simulink subsystem "Point2SHP"  (R2023a)
settings: Solver=VariableStepAuto  StartTime=0.0  StopTime=10.0  RelTol=1e-3
undefined symbols (not defined in the file): magnitude
settings Model: Creator=bjmyn  LastModifiedBy=bjmyn

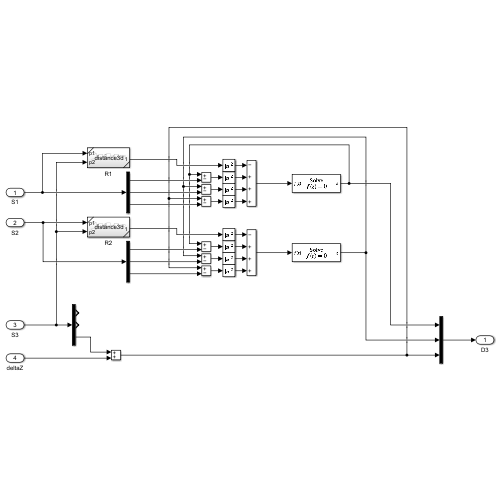
[thumbnail: Simulink's stored preview of the top-level diagram]
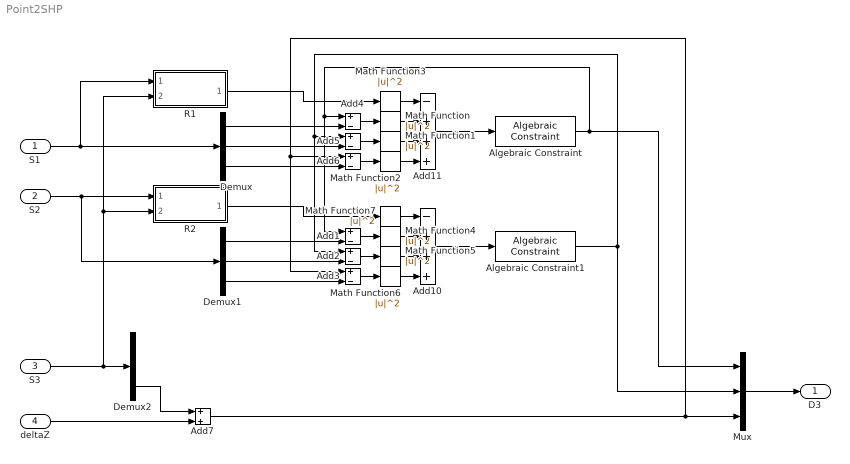
== system Point2SHP ==
  S1 : Inport
  S2 : Inport  Port=2
  S3 : Inport  Port=3
  deltaZ : Inport  Port=4
  Add{1..6} (6 alike) : Sum  Inputs=+-
  Add10 : Sum  Inputs=-+++
  Add11 : Sum  Inputs=-+++
  Add7 : Sum
  Algebraic Constraint : AlgebraicConstraint
  Algebraic Constraint1 : AlgebraicConstraint  InitialGuess=460
  Demux : Demux  Outputs=3
  Demux1 : Demux  Outputs=3
  Demux2 : Demux  Outputs=3
  Math Function{,1..7} (8 alike) : Math  Operator=magnitude^2
  Mux : Mux  Inputs=3
  R1 : Subsystem  ReferencedSubsystem=distance3d
  R2 : Subsystem  ReferencedSubsystem=distance3d
  D3 : Outport
  wires:
  S1/1 -> Demux/1, R1/1
  S3/1 -> Demux2/1, R2/2, R1/2
  Demux1/1 -> Add1/2
  Demux1/2 -> Add2/2
  Demux1/3 -> Add3/2
  Demux/3 -> Add6/2
  Demux/2 -> Add5/2
  Demux/1 -> Add4/2
  Add4/1 -> Math Function/1
  Math Function/1 -> Add11/2
  Math Function1/1 -> Add11/3
  Add5/1 -> Math Function1/1
  Math Function2/1 -> Add11/4
  Add6/1 -> Math Function2/1
  Math Function3/1 -> Add11/1
  R1/1 -> Math Function3/1
  R2/1 -> Math Function7/1
  Math Function7/1 -> Add10/1
  Add3/1 -> Math Function6/1
  Math Function6/1 -> Add10/4
  Add2/1 -> Math Function5/1
  Math Function5/1 -> Add10/3
  Math Function4/1 -> Add10/2
  Add1/1 -> Math Function4/1
  Add11/1 -> Algebraic Constraint/1
  Add10/1 -> Algebraic Constraint1/1
  Mux/1 -> D3/1
  Algebraic Constraint/1 -> Mux/1, Add4/1, Add1/1
  Algebraic Constraint1/1 -> Mux/2, Add5/1, Add2/1
  Add7/1 -> Mux/3, Add6/1, Add3/1
  S2/1 -> Demux1/1, R2/1
  deltaZ/1 -> Add7/2
  Demux2/3 -> Add7/1
